simulink model "PSK (1)"  (R2023b)
settings: Solver=VariableStepAuto  StartTime=0.0  StopTime=10.0  RelTol=1e-3
settings Model: Creator=mluser  LastModifiedBy=mluser

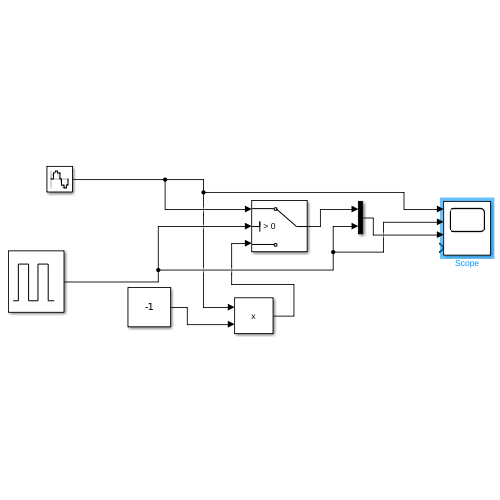
[thumbnail: Simulink's stored preview of the top-level diagram]
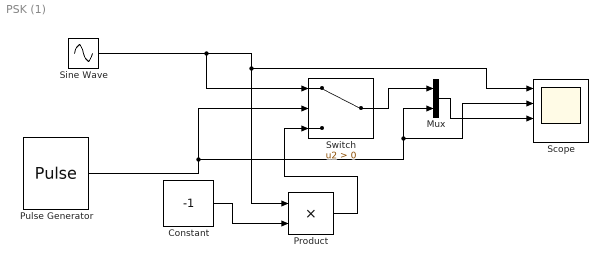
== system PSK (1) ==
  Constant : Constant  Value=-1
  Mux : Mux  Inputs=2
  Product : Product
  Pulse Generator : DiscretePulseGenerator  PulseType=Time based  Period=1  PulseWidth=50
  Scope : Scope  NumInputPorts=4
  Sine Wave : Sin  Frequency=2*pi*2  SampleTime=0.01
  Switch : Switch  Criteria=u2 > Threshold  SaturateOnIntegerOverflow=off  InputSameDT=off
  wires:
  Sine Wave/1 -> Scope/1, Product/1, Switch/1
  Pulse Generator/1 -> Switch/2, Scope/2, Mux/2
  Constant/1 -> Product/2
  Product/1 -> Switch/3
  Switch/1 -> Mux/1
  Mux/1 -> Scope/3
